simulink model "hw3_q10"  (R2019b)
settings: Solver=VariableStepAuto  StartTime=0.0  StopTime=1000  RelTol=1e-3
settings Model: Creator=scjcb  LastModifiedBy=scjcb

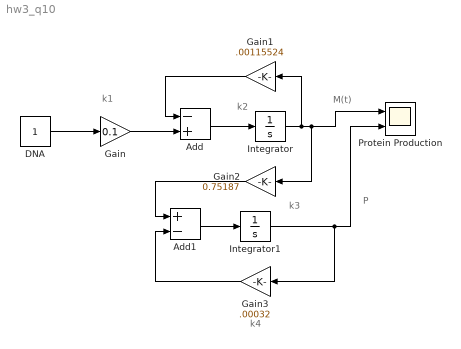
== system hw3_q10 ==
  note: P
  note: M(t)
  note: k1
  note: k4
  note: k3
  note: k2
  Add : Sum  Inputs=-+
  Add1 : Sum  Inputs=+-
  DNA : Constant
  Gain : Gain  Gain=0.1
  Gain1 : Gain  Gain=.00115524
  Gain2 : Gain  Gain=0.75187
  Gain3 : Gain  Gain=.00032
  Integrator : Integrator
  Integrator1 : Integrator
  Protein Production : Scope  NumInputPorts=2
  wires:
  DNA/1 -> Gain/1
  Gain/1 -> Add/2
  Add/1 -> Integrator/1
  Gain1/1 -> Add/1
  Gain2/1 -> Add1/1
  Add1/1 -> Integrator1/1
  Integrator1/1 -> Protein Production/2, Gain3/1
  Gain3/1 -> Add1/2
  Integrator/1 -> Gain1/1, Protein Production/1, Gain2/1
